simulink model "simulationFile"  (R2023a)
settings: Solver=FixedStepAuto  StartTime=0.0  StopTime=50.0  FixedStep=0.005  RelTol=1e-3
PreLoadFcn:
  | run('globalParams.m');
  | global Mode;
  | ProposedController = Simulink.Variant('Mode == 1');
  | ControllerA = Simulink.Variant('Mode == 2');
  | ControllerB = Simulink.Variant('Mode == 3');
settings Model: Creator=Dell Precision  LastModifiedBy=Dell Precision
settings DataIOCC: ReturnWorkspaceOutputs=off

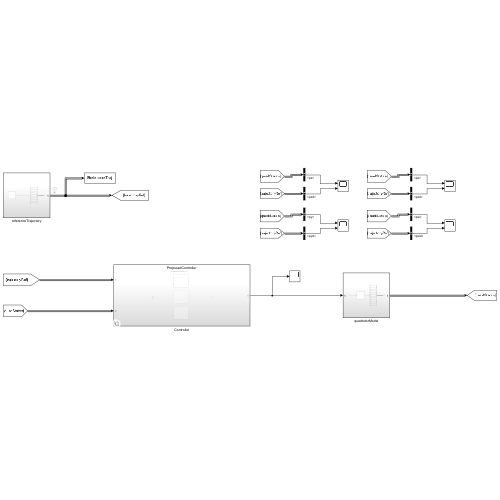
[thumbnail: Simulink's stored preview of the top-level diagram]
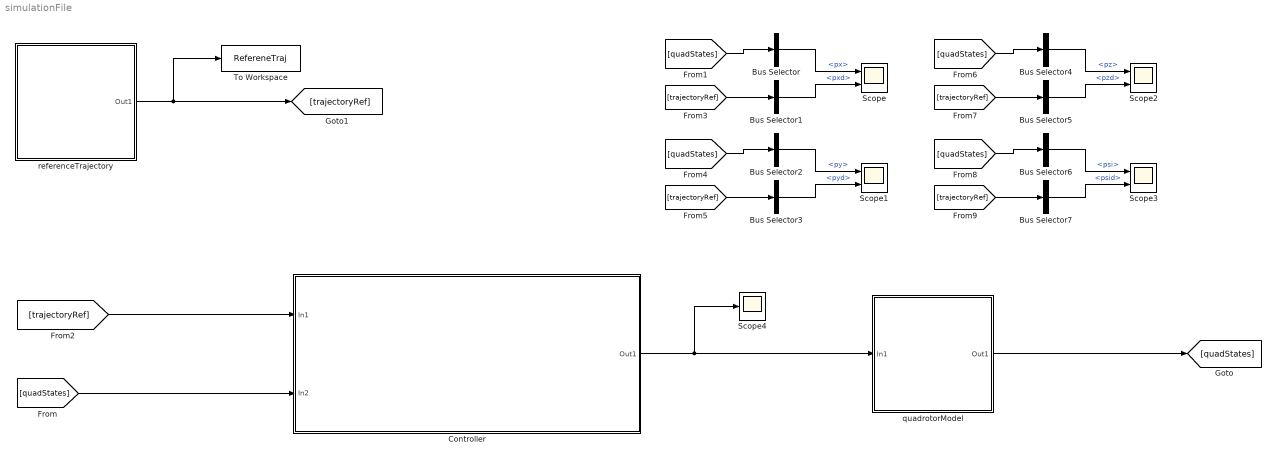
== system simulationFile ==
  Bus Selector : BusSelector  OutputSignals=px
  Bus Selector1 : BusSelector  OutputSignals=pxd
  Bus Selector2 : BusSelector  OutputSignals=py
  Bus Selector3 : BusSelector  OutputSignals=pyd
  Bus Selector4 : BusSelector  OutputSignals=pz
  Bus Selector5 : BusSelector  OutputSignals=pzd
  Bus Selector6 : BusSelector  OutputSignals=psi
  Bus Selector7 : BusSelector  OutputSignals=psid
  Controller : Subsystem  ClipboardFcn=|  Variant=on
      | ProposedController = Simulink.Variant('Mode == 1');
      | ControllerA = Simulink.Variant('Mode == 2');
      | ControllerB = Simulink.Variant('Mode == 3');
      | Mode = 1;
  Scope{,1..3} (4 alike) : Scope  NumInputPorts=2
  Scope4 : Scope
  To Workspace : ToWorkspace  VariableName=RefereneTraj  SaveFormat=Timeseries  SampleTime=-1
  quadrotorModel : Subsystem
  referenceTrajectory : Subsystem
  wires:
  referenceTrajectory/1(Out1) -> To Workspace/1, [trajectoryRef]
  [trajectoryRef] -> Controller/1(In1)
  [quadStates] -> Controller/2(In2)
  Controller/1(Out1) -> quadrotorModel/1(In1), Scope4/1
  [quadStates] -> Bus Selector/1
  [trajectoryRef] -> Bus Selector1/1
  Bus Selector/1 -> Scope/1  "<px>"
  Bus Selector1/1 -> Scope/2  "<pxd>"
  Bus Selector3/1 -> Scope1/2  "<pyd>"
  Bus Selector2/1 -> Scope1/1  "<py>"
  [trajectoryRef] -> Bus Selector3/1
  [quadStates] -> Bus Selector2/1
  [quadStates] -> Bus Selector4/1
  [trajectoryRef] -> Bus Selector5/1
  Bus Selector4/1 -> Scope2/1  "<pz>"
  Bus Selector5/1 -> Scope2/2  "<pzd>"
  Bus Selector7/1 -> Scope3/2  "<psid>"
  Bus Selector6/1 -> Scope3/1  "<psi>"
  [trajectoryRef] -> Bus Selector7/1
  [quadStates] -> Bus Selector6/1
  quadrotorModel/1(Out1) -> [quadStates]

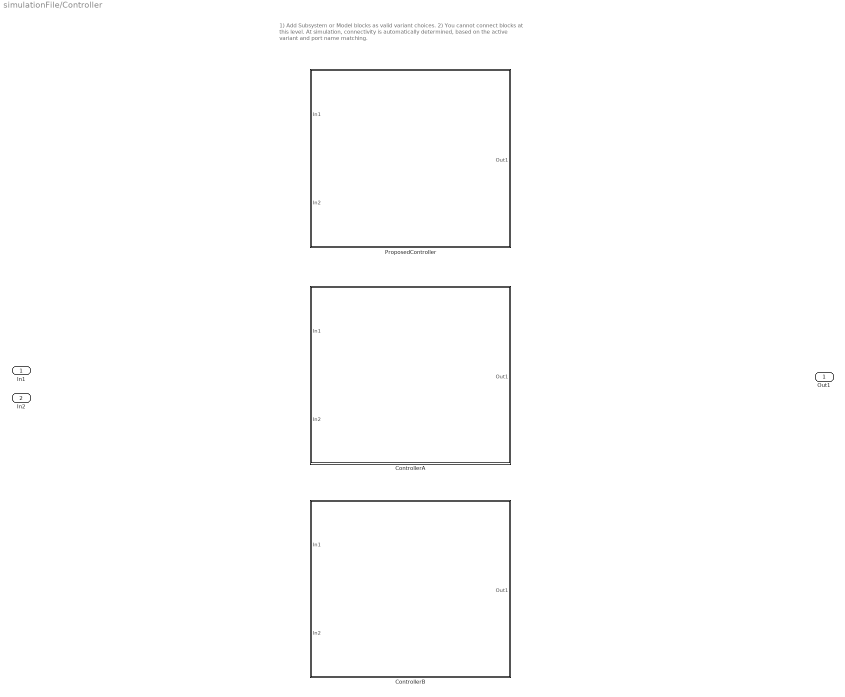
== system simulationFile/Controller ==
  note: 1) Add Subsystem or Model blocks as valid variant choices.
      | 2) You cannot connect blocks at this level. At simulation, connectivity is automatically
      | determined, based on the active variant and port name matching.
  In1 : Inport
  In2 : Inport  Port=2
  ControllerA : Subsystem  VariantControl=ControllerA
  ControllerB : Subsystem  VariantControl=ControllerB
  ProposedController : Subsystem  VariantControl=ProposedController
  Out1 : Outport

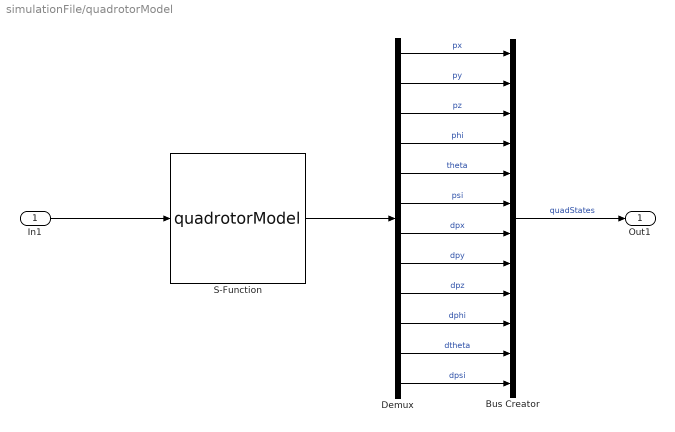
== system simulationFile/quadrotorModel ==
  In1 : Inport
  Bus Creator : BusCreator  Inputs=12
  Demux : Demux  Outputs=12
  S-Function : S-Function  FunctionName=quadrotorModel  SFunctionDeploymentMode=off  EnableBusSupport=off
  Out1 : Outport
  wires:
  In1/1 -> S-Function/1
  S-Function/1 -> Demux/1
  Demux/1 -> Bus Creator/1  "px"
  Demux/8 -> Bus Creator/8  "dpy"
  Demux/9 -> Bus Creator/9  "dpz"
  Demux/10 -> Bus Creator/10  "dphi"
  Demux/11 -> Bus Creator/11  "dtheta"
  Demux/12 -> Bus Creator/12  "dpsi"
  Demux/2 -> Bus Creator/2  "py"
  Demux/3 -> Bus Creator/3  "pz"
  Demux/4 -> Bus Creator/4  "phi"
  Demux/5 -> Bus Creator/5  "theta"
  Demux/6 -> Bus Creator/6  "psi"
  Demux/7 -> Bus Creator/7  "dpx"
  Bus Creator/1 -> Out1/1  "quadStates"

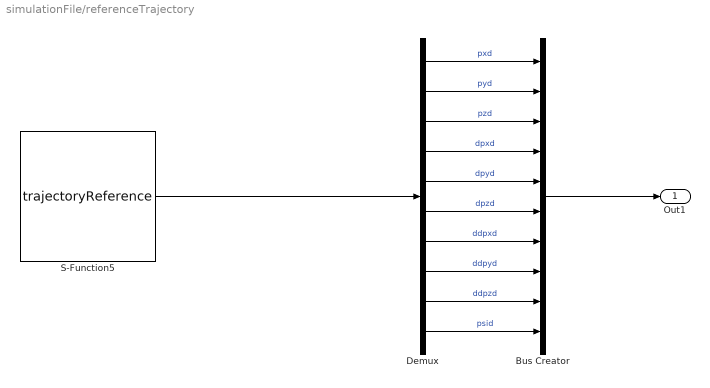
== system simulationFile/referenceTrajectory ==
  Bus Creator : BusCreator  Inputs=10
  Demux : Demux  Outputs=10
  S-Function5 : S-Function  FunctionName=trajectoryReference  SFunctionDeploymentMode=off  EnableBusSupport=off
  Out1 : Outport
  wires:
  Demux/7 -> Bus Creator/7  "ddpxd"
  Demux/8 -> Bus Creator/8  "ddpyd"
  Demux/9 -> Bus Creator/9  "ddpzd"
  Demux/1 -> Bus Creator/1  "pxd"
  Demux/2 -> Bus Creator/2  "pyd"
  Demux/3 -> Bus Creator/3  "pzd"
  Demux/4 -> Bus Creator/4  "dpxd"
  Demux/5 -> Bus Creator/5  "dpyd"
  Demux/6 -> Bus Creator/6  "dpzd"
  Bus Creator/1 -> Out1/1
  Demux/10 -> Bus Creator/10  "psid"
  S-Function5/1 -> Demux/1

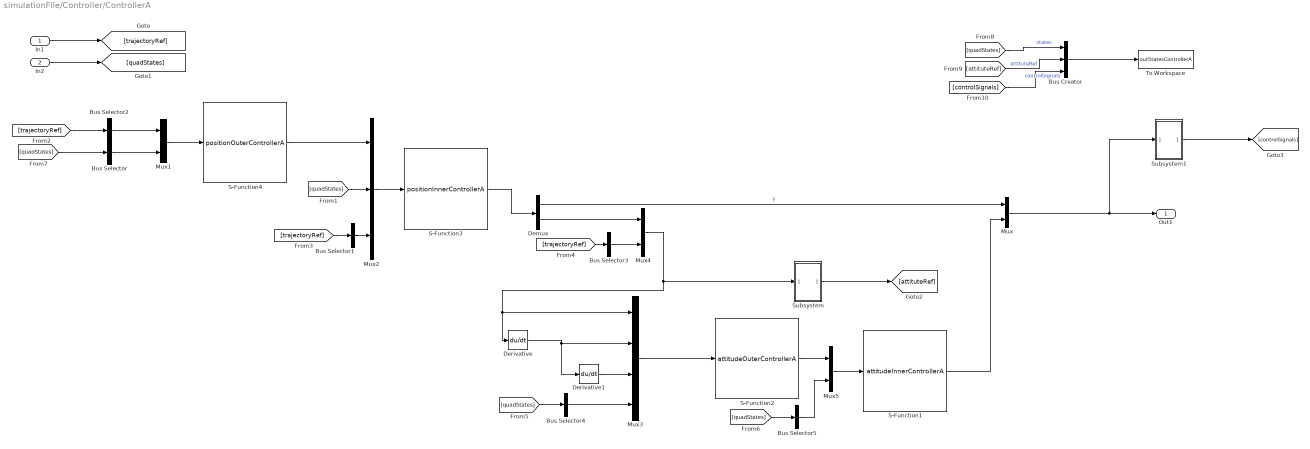
== system simulationFile/Controller/ControllerA ==
  In1 : Inport
  In2 : Inport  Port=2
  Bus Creator : BusCreator  Inputs=3
  Bus Selector : BusSelector  OutputSignals=px,py,pz,dpx,dpy,dpz  OutputAsBus=on
  Bus Selector1 : BusSelector  OutputSignals=ddpxd,ddpyd,ddpzd,psid  OutputAsBus=on
  Bus Selector2 : BusSelector  OutputSignals=pxd,pyd,pzd,dpxd,dpyd,dpzd,ddpxd,ddpyd,ddpzd  OutputAsBus=on
  Bus Selector3 : BusSelector  OutputSignals=psid  OutputAsBus=on
  Bus Selector4 : BusSelector  OutputSignals=phi,theta,psi,dphi,dtheta,dpsi  OutputAsBus=on
  Bus Selector5 : BusSelector  OutputSignals=phi,theta,psi,dphi,dtheta,dpsi  OutputAsBus=on
  Demux : Demux  Outputs=[1,2]
  Derivative : Derivative
  Derivative1 : Derivative
  Mux{,1,4..5} (4 alike) : Mux  Inputs=2
  Mux2 : Mux  Inputs=3
  Mux3 : Mux
  S-Function1 : S-Function  FunctionName=attitudeInnerControllerA  SFunctionDeploymentMode=off  EnableBusSupport=off
  S-Function2 : S-Function  FunctionName=attitudeOuterControllerA  SFunctionDeploymentMode=off  EnableBusSupport=off
  S-Function3 : S-Function  FunctionName=positionInnerControllerA  SFunctionDeploymentMode=off  EnableBusSupport=off
  S-Function4 : S-Function  FunctionName=positionOuterControllerA  SFunctionDeploymentMode=off  EnableBusSupport=off
  Subsystem : Subsystem
  Subsystem1 : Subsystem
  To Workspace : ToWorkspace  VariableName=outStatesControllerA  SaveFormat=Timeseries  SampleTime=-1
  Out1 : Outport
  wires:
  Derivative1/1 -> Mux3/3
  Demux/1 -> Mux/1  "F"
  S-Function2/1 -> Mux5/1
  Mux5/1 -> S-Function1/1
  Mux2/1 -> S-Function3/1
  S-Function4/1 -> Mux2/1
  Bus Selector4/1 -> Mux3/4
  S-Function3/1 -> Demux/1
  Bus Selector3/1 -> Mux4/2
  [trajectoryRef] -> Bus Selector3/1
  Bus Selector5/1 -> Mux5/2
  [quadStates] -> Bus Selector5/1
  Derivative/1 -> Mux3/2, Derivative1/1
  Mux3/1 -> S-Function2/1
  Demux/2 -> Mux4/1
  S-Function1/1 -> Mux/2
  Mux1/1 -> S-Function4/1
  Bus Selector/1 -> Mux1/2
  Bus Selector1/1 -> Mux2/3
  Bus Selector2/1 -> Mux1/1
  [trajectoryRef] -> Bus Selector1/1
  [quadStates] -> Bus Selector4/1
  [quadStates] -> Mux2/2
  In1/1 -> [trajectoryRef]
  In2/1 -> [quadStates]
  [trajectoryRef] -> Bus Selector2/1
  [quadStates] -> Bus Selector/1
  [attituteRef] -> Bus Creator/2  "attituteRef"
  [controlSignals] -> Bus Creator/3  "controlSignals"
  [quadStates] -> Bus Creator/1  "states"
  Bus Creator/1 -> To Workspace/1
  Mux4/1 -> Subsystem/1(In1), Mux3/1, Derivative/1
  Subsystem/1(Out1) -> [attituteRef]
  Subsystem1/1(Out1) -> [controlSignals]
  Mux/1 -> Subsystem1/1(In1), Out1/1

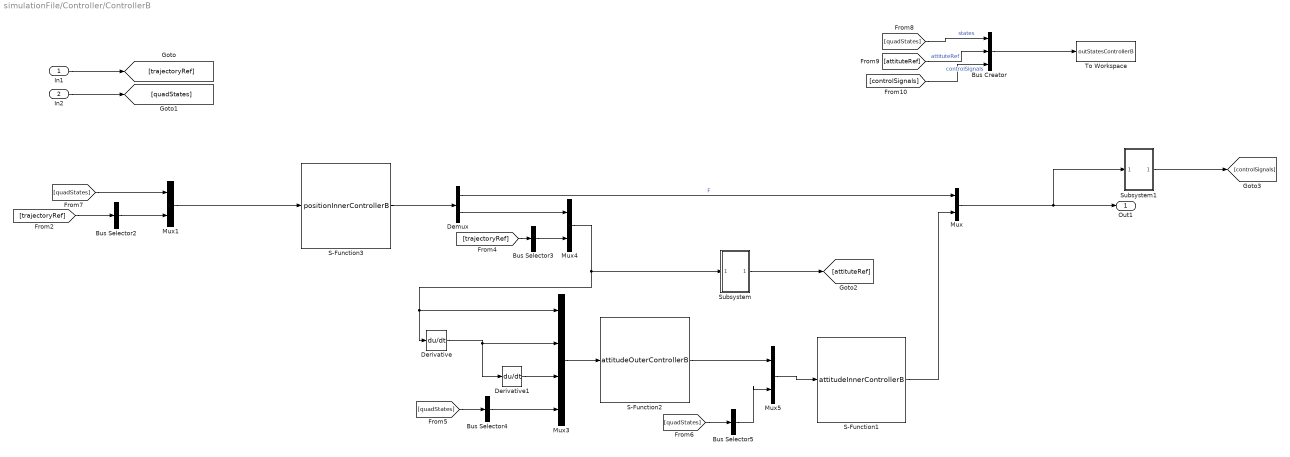
== system simulationFile/Controller/ControllerB ==
  In1 : Inport
  In2 : Inport  Port=2
  Bus Creator : BusCreator  Inputs=3
  Bus Selector2 : BusSelector  OutputSignals=pxd,pyd,pzd,dpxd,dpyd,dpzd,ddpxd,ddpyd,ddpzd,psid  OutputAsBus=on
  Bus Selector3 : BusSelector  OutputSignals=psid  OutputAsBus=on
  Bus Selector4 : BusSelector  OutputSignals=phi,theta,psi,dphi,dtheta,dpsi  OutputAsBus=on
  Bus Selector5 : BusSelector  OutputSignals=phi,theta,psi,dphi,dtheta,dpsi  OutputAsBus=on
  Demux : Demux  Outputs=[1,2]
  Derivative : Derivative
  Derivative1 : Derivative
  Mux{,1,4..5} (4 alike) : Mux  Inputs=2
  Mux3 : Mux
  S-Function1 : S-Function  FunctionName=attitudeInnerControllerB  SFunctionDeploymentMode=off  EnableBusSupport=off
  S-Function2 : S-Function  FunctionName=attitudeOuterControllerB  SFunctionDeploymentMode=off  EnableBusSupport=off
  S-Function3 : S-Function  FunctionName=positionInnerControllerB  SFunctionDeploymentMode=off  EnableBusSupport=off
  Subsystem : Subsystem
  Subsystem1 : Subsystem
  To Workspace : ToWorkspace  VariableName=outStatesControllerB  SaveFormat=Timeseries  SampleTime=-1
  Out1 : Outport
  wires:
  [trajectoryRef] -> Bus Selector2/1
  In2/1 -> [quadStates]
  In1/1 -> [trajectoryRef]
  [quadStates] -> Bus Selector4/1
  Mux1/1 -> S-Function3/1
  S-Function1/1 -> Mux/2
  Demux/2 -> Mux4/1
  Mux3/1 -> S-Function2/1
  Derivative/1 -> Derivative1/1, Mux3/2
  [quadStates] -> Bus Selector5/1
  Bus Selector5/1 -> Mux5/2
  [trajectoryRef] -> Bus Selector3/1
  Bus Selector3/1 -> Mux4/2
  S-Function3/1 -> Demux/1
  Bus Selector4/1 -> Mux3/4
  Mux5/1 -> S-Function1/1
  S-Function2/1 -> Mux5/1
  Demux/1 -> Mux/1  "F"
  Derivative1/1 -> Mux3/3
  Bus Selector2/1 -> Mux1/2
  [quadStates] -> Mux1/1
  [attituteRef] -> Bus Creator/2  "attituteRef"
  [controlSignals] -> Bus Creator/3  "controlSignals"
  [quadStates] -> Bus Creator/1  "states"
  Bus Creator/1 -> To Workspace/1
  Mux4/1 -> Subsystem/1(In1), Derivative/1, Mux3/1
  Subsystem/1(Out1) -> [attituteRef]
  Subsystem1/1(Out1) -> [controlSignals]
  Mux/1 -> Subsystem1/1(In1), Out1/1

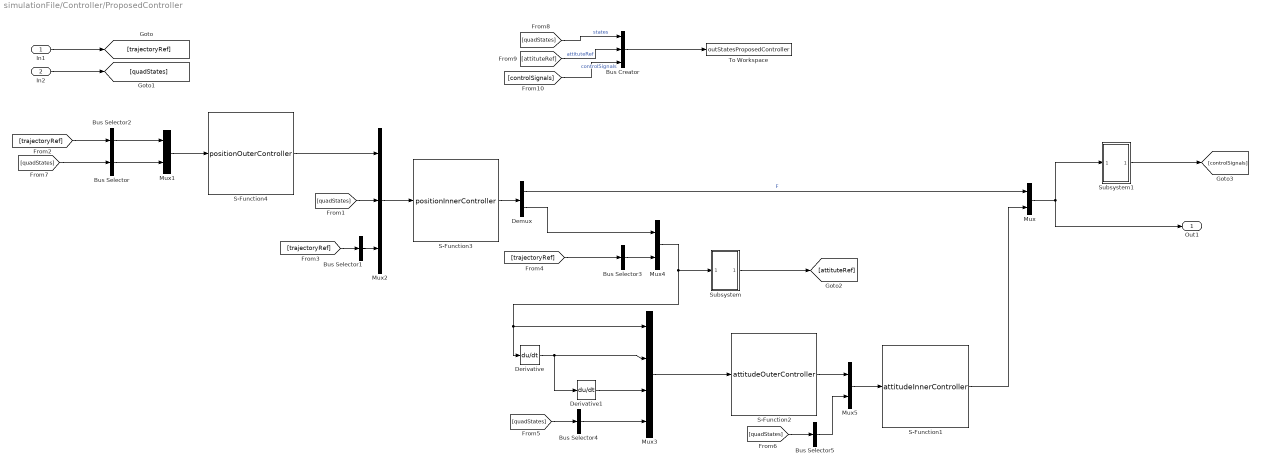
== system simulationFile/Controller/ProposedController ==
  In1 : Inport
  In2 : Inport  Port=2
  Bus Creator : BusCreator  Inputs=3
  Bus Selector : BusSelector  OutputSignals=px,py,pz,dpx,dpy,dpz  OutputAsBus=on
  Bus Selector1 : BusSelector  OutputSignals=ddpxd,ddpyd,ddpzd,psid  OutputAsBus=on
  Bus Selector2 : BusSelector  OutputSignals=pxd,pyd,pzd,dpxd,dpyd,dpzd,ddpxd,ddpyd,ddpzd  OutputAsBus=on
  Bus Selector3 : BusSelector  OutputSignals=psid  OutputAsBus=on
  Bus Selector4 : BusSelector  OutputSignals=phi,theta,psi,dphi,dtheta,dpsi  OutputAsBus=on
  Bus Selector5 : BusSelector  OutputSignals=phi,theta,psi,dphi,dtheta,dpsi  OutputAsBus=on
  Demux : Demux  Outputs=[1,2]
  Derivative : Derivative
  Derivative1 : Derivative
  Mux{,1,4..5} (4 alike) : Mux  Inputs=2
  Mux2 : Mux  Inputs=3
  Mux3 : Mux
  S-Function1 : S-Function  FunctionName=attitudeInnerController  SFunctionDeploymentMode=off  EnableBusSupport=off
  S-Function2 : S-Function  FunctionName=attitudeOuterController  SFunctionDeploymentMode=off  EnableBusSupport=off
  S-Function3 : S-Function  FunctionName=positionInnerController  SFunctionDeploymentMode=off  EnableBusSupport=off
  S-Function4 : S-Function  FunctionName=positionOuterController  SFunctionDeploymentMode=off  EnableBusSupport=off
  Subsystem : Subsystem
  Subsystem1 : Subsystem
  To Workspace : ToWorkspace  VariableName=outStatesProposedController  SaveFormat=Timeseries  SampleTime=-1
  Out1 : Outport
  wires:
  [quadStates] -> Mux2/2
  [quadStates] -> Bus Selector4/1
  [trajectoryRef] -> Bus Selector1/1
  Bus Selector1/1 -> Mux2/3
  S-Function1/1 -> Mux/2
  Demux/2 -> Mux4/1
  Mux3/1 -> S-Function2/1
  Mux4/1 -> Subsystem/1(In1), Derivative/1, Mux3/1
  Derivative/1 -> Mux3/2, Derivative1/1
  [quadStates] -> Bus Selector5/1
  Bus Selector5/1 -> Mux5/2
  [trajectoryRef] -> Bus Selector3/1
  Bus Selector3/1 -> Mux4/2
  S-Function3/1 -> Demux/1
  Bus Selector4/1 -> Mux3/4
  S-Function4/1 -> Mux2/1
  Mux2/1 -> S-Function3/1
  Mux5/1 -> S-Function1/1
  S-Function2/1 -> Mux5/1
  Demux/1 -> Mux/1  "F"
  Derivative1/1 -> Mux3/3
  [quadStates] -> Bus Selector/1
  Bus Selector2/1 -> Mux1/1
  In2/1 -> [quadStates]
  Bus Selector/1 -> Mux1/2
  [trajectoryRef] -> Bus Selector2/1
  Mux1/1 -> S-Function4/1
  In1/1 -> [trajectoryRef]
  [quadStates] -> Bus Creator/1  "states"
  Subsystem/1(Out1) -> [attituteRef]
  [attituteRef] -> Bus Creator/2  "attituteRef"
  Bus Creator/1 -> To Workspace/1
  Subsystem1/1(Out1) -> [controlSignals]
  Mux/1 -> Out1/1, Subsystem1/1(In1)
  [controlSignals] -> Bus Creator/3  "controlSignals"

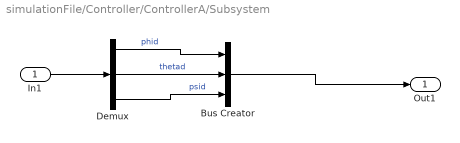
== system simulationFile/Controller/ControllerA/Subsystem ==
  In1 : Inport
  Bus Creator : BusCreator  Inputs=3
  Demux : Demux  Outputs=3
  Out1 : Outport
  wires:
  Bus Creator/1 -> Out1/1
  Demux/1 -> Bus Creator/1  "phid"
  Demux/2 -> Bus Creator/2  "thetad"
  Demux/3 -> Bus Creator/3  "psid"
  In1/1 -> Demux/1

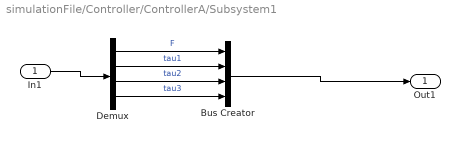
== system simulationFile/Controller/ControllerA/Subsystem1 ==
  In1 : Inport
  Bus Creator : BusCreator  Inputs=4
  Demux : Demux
  Out1 : Outport
  wires:
  In1/1 -> Demux/1
  Demux/3 -> Bus Creator/3  "tau2"
  Demux/2 -> Bus Creator/2  "tau1"
  Demux/1 -> Bus Creator/1  "F"
  Bus Creator/1 -> Out1/1
  Demux/4 -> Bus Creator/4  "tau3"

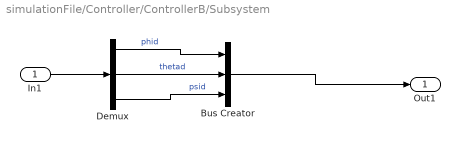
== system simulationFile/Controller/ControllerB/Subsystem ==
  In1 : Inport
  Bus Creator : BusCreator  Inputs=3
  Demux : Demux  Outputs=3
  Out1 : Outport
  wires:
  Bus Creator/1 -> Out1/1
  Demux/1 -> Bus Creator/1  "phid"
  Demux/2 -> Bus Creator/2  "thetad"
  Demux/3 -> Bus Creator/3  "psid"
  In1/1 -> Demux/1

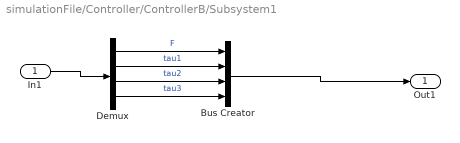
== system simulationFile/Controller/ControllerB/Subsystem1 ==
  In1 : Inport
  Bus Creator : BusCreator  Inputs=4
  Demux : Demux
  Out1 : Outport
  wires:
  In1/1 -> Demux/1
  Demux/3 -> Bus Creator/3  "tau2"
  Demux/2 -> Bus Creator/2  "tau1"
  Demux/1 -> Bus Creator/1  "F"
  Bus Creator/1 -> Out1/1
  Demux/4 -> Bus Creator/4  "tau3"

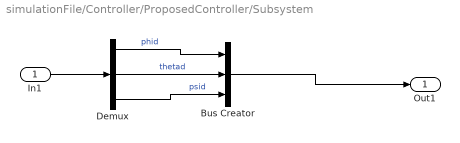
== system simulationFile/Controller/ProposedController/Subsystem ==
  In1 : Inport
  Bus Creator : BusCreator  Inputs=3
  Demux : Demux  Outputs=3
  Out1 : Outport
  wires:
  Bus Creator/1 -> Out1/1
  Demux/1 -> Bus Creator/1  "phid"
  Demux/2 -> Bus Creator/2  "thetad"
  Demux/3 -> Bus Creator/3  "psid"
  In1/1 -> Demux/1

== system simulationFile/Controller/ProposedController/Subsystem1 ==
  In1 : Inport
  Bus Creator : BusCreator  Inputs=4
  Demux : Demux
  Out1 : Outport
  wires:
  In1/1 -> Demux/1
  Demux/3 -> Bus Creator/3  "tau2"
  Demux/2 -> Bus Creator/2  "tau1"
  Demux/1 -> Bus Creator/1  "F"
  Bus Creator/1 -> Out1/1
  Demux/4 -> Bus Creator/4  "tau3"
